simulink model "LuGre_model_A"  (R2026a)
settings: Solver=ode15s  StopTime=14  MaxStep=1e-5  RelTol=1e-7
settings Model: NumberOfSteps=10  Creator=kikuchi  LastModifiedBy=kikuchi

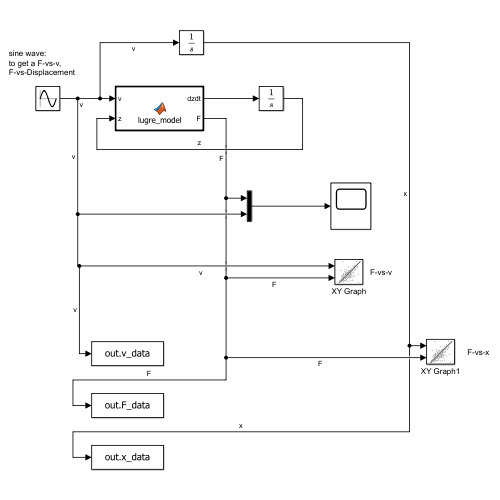
[thumbnail: Simulink's stored preview of the top-level diagram]
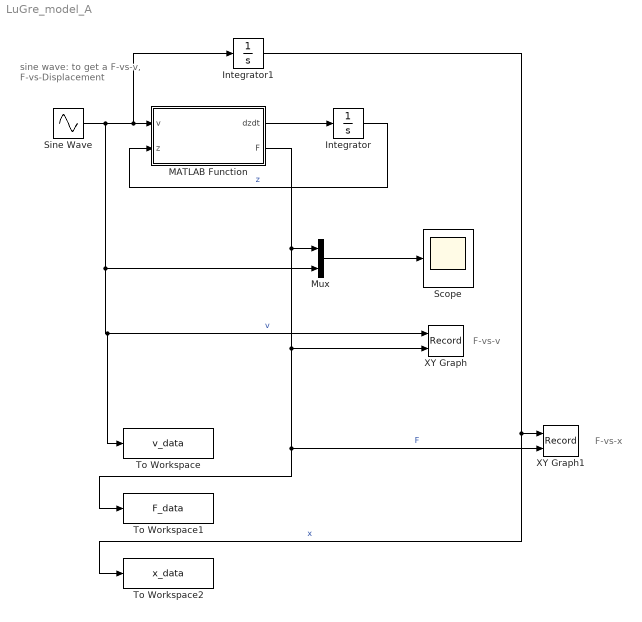
== system LuGre_model_A ==
  note: sine wave:
      | to get a F-vs-v,
      | F-vs-Displacement
  note: F-vs-v
  note: F-vs-x
  Integrator : Integrator
  Integrator1 : Integrator
  MATLAB Function : MATLAB Function  TreatAsAtomicUnit=on
  Mux : Mux  Inputs=2
  Scope : Scope
      settings: ActiveDisplayYMinimum=-7.5445326454646242  ActiveDisplayYMaximum=4.8434715839579514
  Sine Wave : Sin  Amplitude=1e-4  Frequency=0.6  SampleTime=0
  To Workspace : ToWorkspace  VariableName=v_data  SampleTime=-1
  To Workspace1 : ToWorkspace  VariableName=F_data  SampleTime=-1
  To Workspace2 : ToWorkspace  VariableName=x_data  SampleTime=-1
  XY Graph : Record  NumPorts=2.0  FileSettingsInternal="{\"entries\":[{\"content\":{\"excelSettings\":{\"content\":{},\"type\":\"Streamout.ExcelSettings\"},\"parquetSettings\":{\"content\":{},\"type\":\"Streamout.ParquetSettings\"}},\"type\":\"Streamout.FileSettingStorage\",\"uuid\":\"\"}],\"packageUris\":[\"http:\\/\\/schema.mathworks.com\\/mf0\\/streamout_blocks\\/R2020a\"],\"version\":\"1.0\"}"  FrameSettings=[0, 0]  Layout=[1 1]  SignalsInternal="{\"entries\":[{\"content\":{\"signals\":[{\"content\":{\"blockPath\":[],\"dimensions\":[1],\"domain\":\"\",\"lineColor\":\"#a2142f\",\"plots\":[ 1 ],\"port\":1,\"sid\":[\"\"],\"signalID\":1,\"signalName\":\"v\"},\"type\":\"RecordBlkView.Signal\",\"uuid\":\"\"},{\"content\":{\"blockPath\":[],\"dimensions\":[1],\"domain\":\"\",\"lineColor\":\"#139fff\",\"plots\":[ 1 ],\"port\":2,\"sid\":[\"\"],\"signalID\":2,\"signalName\":\"F\"},\"type\":\"RecordBlkView.Signal\",\"uuid\":\"\"}]},\"type\":\"RecordBlkView.InputSignals\",\"uuid\":\"\"}],\"packageUris\":[\"http:\\/\\/schema.mathworks.com\\/mf0\\/streamout_blocks\\/R2020a\"],\"version\":\"1.0\"}"  VisualizationBindings="{\"xyplotplugin\":{\"info\":[{\"series\":[{\"bindingParametersList\":[{\"parameter\":\"X-Axis\",\"signalID\":1,\"signalName\":\"v\"},{\"parameter\":\"Y-Axis\",\"signalID\":2,\"signalName\":\"F\"}],\"seriesID\":0}],\"subplotID\":1}]}}"  CompatibilityTag=XY
  XY Graph1 : Record  NumPorts=2.0  FileSettingsInternal="{\"entries\":[{\"content\":{\"excelSettings\":{\"content\":{},\"type\":\"Streamout.ExcelSettings\"},\"parquetSettings\":{\"content\":{},\"type\":\"Streamout.ParquetSettings\"}},\"type\":\"Streamout.FileSettingStorage\",\"uuid\":\"\"}],\"packageUris\":[\"http:\\/\\/schema.mathworks.com\\/mf0\\/streamout_blocks\\/R2020a\"],\"version\":\"1.0\"}"  FrameSettings=[0, 0]  Layout=[1 1]  SignalsInternal="{\"entries\":[{\"content\":{\"signals\":[{\"content\":{\"blockPath\":[],\"dimensions\":[1],\"domain\":\"\",\"lineColor\":\"#a2142f\",\"plots\":[ 1 ],\"port\":1,\"sid\":[\"\"],\"signalID\":1,\"signalName\":\"x\"},\"type\":\"RecordBlkView.Signal\",\"uuid\":\"\"},{\"content\":{\"blockPath\":[],\"dimensions\":[1],\"domain\":\"\",\"lineColor\":\"#139fff\",\"plots\":[ 1 ],\"port\":2,\"sid\":[\"\"],\"signalID\":2,\"signalName\":\"F\"},\"type\":\"RecordBlkView.Signal\",\"uuid\":\"\"}]},\"type\":\"RecordBlkView.InputSignals\",\"uuid\":\"\"}],\"packageUris\":[\"http:\\/\\/schema.mathworks.com\\/mf0\\/streamout_blocks\\/R2020a\"],\"version\":\"1.0\"}"  VisualizationBindings="{\"xyplotplugin\":{\"info\":[{\"series\":[{\"bindingParametersList\":[{\"parameter\":\"X-Axis\",\"signalID\":1,\"signalName\":\"x\"},{\"parameter\":\"Y-Axis\",\"signalID\":2,\"signalName\":\"F\"}],\"seriesID\":0}],\"subplotID\":1}]}}"  CompatibilityTag=XY
  wires:
  Sine Wave/1 -> Integrator1/1, MATLAB Function/1(v), To Workspace/1, XY Graph/1, Mux/2  "v"
  MATLAB Function/1(dzdt) -> Integrator/1
  Integrator/1 -> MATLAB Function/2(z)  "z"
  MATLAB Function/2(F) -> XY Graph1/2, To Workspace1/1, XY Graph/2, Mux/1  "F"
  Mux/1 -> Scope/1
  Integrator1/1 -> To Workspace2/1, XY Graph1/1  "x"

== matlab function LuGre_model_A/MATLAB Function ==
  data: v input; dzdt output; z input; F output
function [dzdt, F] = lugre_model(v, z)
    % parameters (from the table I in the paper of LuGre) 
    sigma0 = 1e5; % stiffness, refined
    sigma1 = sqrt(sigma0) % damping(減衰)
    sigma2 = 0.4; % viscosity coefficient(粘性係数)
    Fc = 1.0; % dynamic friction force(動摩擦力)
    Fs = 1.5; % static friction force(静止摩擦力)
    vs = 0.001; % stribeck speed(ストライベック速度)
    
    % g(v)
    gv = Fc + (Fs - Fc) * exp(-(v/vs)^2);
    
    % dz/dt
    dzdt = v - (sigma0 * abs(v) / gv) * z;
    
    % F
    F = sigma0 * z + sigma1 * dzdt + sigma2 * v;
end
